simulink model "dsbscfinal"  (R2021b)
settings: Solver=ode45  StartTime=0.0  StopTime=2  RelTol=1e-3  EnableMultiTasking=on
libraries: dsparch4 x1
settings Model: Creator=dhairya  LastModifiedBy=91934
settings SolverCC: AlgebraicLoopSolver=TrustRegion
settings DataIOCC: LimitDataPoints=on  SaveFormat=Array  ReturnWorkspaceOutputs=off
settings OptimizationCC: LifeSpan=inf
settings DebuggingCC: SFUnexpectedBacktrackingDiag=warning  SFNoUnconditionalDefaultTransitionDiag=warning  SFExecutionAtInitializationDiag=none  SFMachineParentedDataDiag=warning  ArithmeticOperatorsInVariantConditions=warning
settings HardwareCC: ProdBitPerPointer=32  ProdBitPerSizeT=32  ProdBitPerPtrDiffT=32  ProdLargestAtomicFloat=None  ProdIntDivRoundTo=Undefined  ProdEndianess=Unspecified  ProdWordSize=32  ProdHWDeviceType=32-bit Generic
settings ModelReferenceCC: PropagateSignalLabelsOutOfModel=off
settings SFSimCC: SimUseLocalCustomCode=off  CustomCodeUndefinedFunction=UseInterfaceOnly
settings RTWCC: RTWUseLocalCustomCode=off
settings CodeAppCC: StateflowObjectComments=on
settings GRTTargetCC: TargetLangStandard=C89/C90 (ANSI)
settings ConfigComp: CovMetricSettings=dw  CovSaveCumulativeToWorkspaceVar=on  CovSaveSingleToWorkspaceVar=on  CovExternalEMLEnable=off

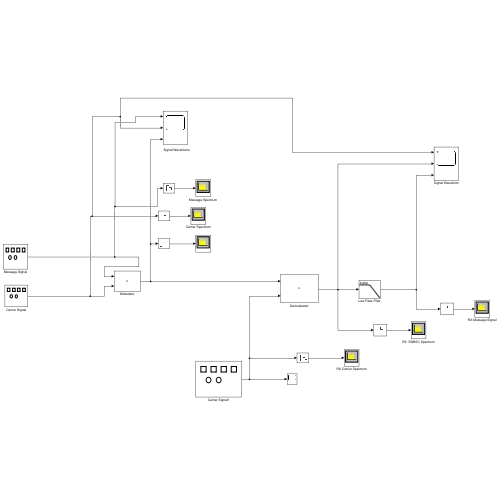
[thumbnail: Simulink's stored preview of the top-level diagram]
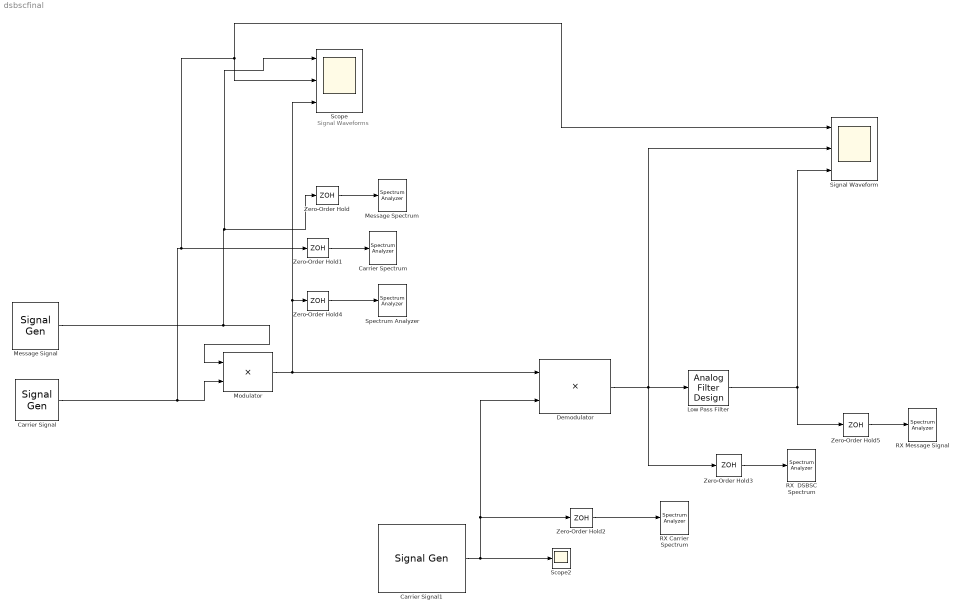
== system dsbscfinal ==
  note: Signal Waveforms
  Carrier Signal : SignalGenerator  Frequency=1500
  Carrier Signal1 : SignalGenerator  Frequency=1500
  Carrier Spectrum : SpectrumAnalyzer
  Demodulator : Product
  Low Pass Filter : dsparch4/Analog Filter Design  method=Butterworth  filttype=Lowpass  N=8  Wlo=2*pi*400  Whi=80  Rp=2  Rs=40
  Message Signal : SignalGenerator  Frequency=100
  Message Spectrum : SpectrumAnalyzer
  Modulator : Product
  RX  DSBSC Spectrum : SpectrumAnalyzer
  RX Carrier Spectrum : SpectrumAnalyzer
  RX Message Signal : SpectrumAnalyzer
  Scope : Scope  NumInputPorts=3
  Scope2 : Scope
  Signal Waveform : Scope  NumInputPorts=3
  Spectrum Analyzer : SpectrumAnalyzer
  Zero-Order Hold : ZeroOrderHold  SampleTime=1/4000
  Zero-Order Hold{1..3,5} (4 alike) : ZeroOrderHold  SampleTime=1/30000
  Zero-Order Hold4 : ZeroOrderHold  SampleTime=-1
  wires:
  Zero-Order Hold/1 -> Message Spectrum/1
  Zero-Order Hold1/1 -> Carrier Spectrum/1
  Zero-Order Hold2/1 -> RX Carrier Spectrum/1
  Carrier Signal1/1 -> Demodulator/2, Zero-Order Hold2/1, Scope2/1
  Zero-Order Hold5/1 -> RX Message Signal/1
  Low Pass Filter/1 -> Zero-Order Hold5/1, Signal Waveform/3
  Demodulator/1 -> Signal Waveform/2, Zero-Order Hold3/1, Low Pass Filter/1
  Zero-Order Hold4/1 -> Spectrum Analyzer/1
  Modulator/1 -> Scope/3, Zero-Order Hold4/1, Demodulator/1
  Message Signal/1 -> Modulator/1, Scope/1, Zero-Order Hold/1
  Zero-Order Hold3/1 -> RX  DSBSC Spectrum/1
  Carrier Signal/1 -> Scope/2, Signal Waveform/1, Zero-Order Hold1/1, Modulator/2
